simulink model "Copy_ofCorrecteurReel"  (R2020a)
settings: Solver=FixedStepDiscrete  StartTime=0.0  StopTime=10  FixedStep=Te  RelTol=1e-3
undefined symbols (not defined in the file or in its folder): National_Instruments, PCI, PID1, Te
libraries: sldrtlib x2
settings Model: Creator=garnica-aza  LastModifiedBy=garnica-aza
settings OptimizationCC: DefaultParameterBehavior=Inlined  EnhancedBackFolding=on  PassReuseOutputArgsThreshold=0  OptimizeBlockOrder=speed  DifferentSizesBufferReuse=on  OptimizationCustomize=off
settings DebuggingCC: ParameterTunabilityLossMsg=error
settings SFSimCC: MATLABDynamicMemAlloc=off
settings RTWCC: Description=Simulink Desktop Real-Time  SystemTargetFile=sldrt.tlc  TemplateMakefile=sldrt.tmf  RTWCompilerOptimization=on
settings CodeAppCC: ForceParamTrailComments=on  MaxIdLength=95  OperatorAnnotations=on
settings SimulinkDesktopRealTimeCC: TargetPreCompLibLocation=C:\Program Files\MATLAB\R2020a\toolbox\sldrt\lib\win64

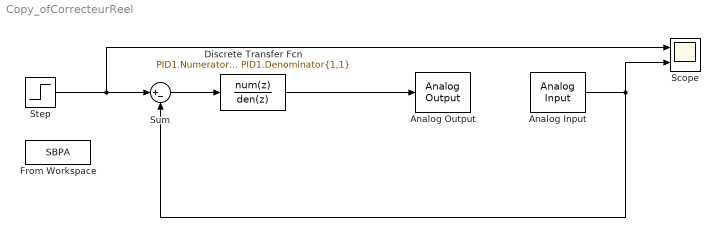
== system Copy_ofCorrecteurReel ==
  Analog Input : sldrtlib/Analog Input  SampleTime=Te  MaxMissedTicks=10  ShowMissedTicks=off  YieldWhenWaiting=off  DrvName=National_Instruments/PCI-6024E  DrvAddress=4294967295  DrvOptions=[0 0 0 0 0 0]  Channels=1  RangeMode=1  VoltRange=1  DataType=1
      settings: AttributesFormatString=National Instruments\nPCI-6024E [auto]
  Analog Output : sldrtlib/Analog Output  SampleTime=Te  MaxMissedTicks=10  ShowMissedTicks=off  YieldWhenWaiting=off  DrvName=National_Instruments/PCI-6024E  DrvAddress=4294967295  DrvOptions=[0 0 0 0 0 0]  Channels=1  RangeMode=1  VoltRange=1  InitialValue=0  FinalValue=0
      settings: AttributesFormatString=National Instruments\nPCI-6024E [auto]
  Discrete Transfer Fcn : DiscreteTransferFcn  Numerator=PID1.Numerator{1,1}  Denominator=PID1.Denominator{1,1}
  From Workspace : FromWorkspace  VariableName=SBPA
  Scope : Scope  NumInputPorts=2
  Step : Step  After=3  SampleTime=0
  Sum : Sum  Inputs=|+-
  wires:
  Analog Input/1 -> Sum/2, Scope/2
  Discrete Transfer Fcn/1 -> Analog Output/1
  Sum/1 -> Discrete Transfer Fcn/1
  Step/1 -> Scope/1, Sum/1
